simulink model "RealLifeTrainModel"  (R2024a)
settings: Solver=ode1  StartTime=0.0  StopTime=Inf  FixedStep=0.001  RelTol=1e-3
PostLoadFcn:
  | , if any(exist('dsrtsu_mdlpostloadfcn', 'file') ~= 0), dsrtsu_mdlpostloadfcn('Execute', bdroot); end,
InitFcn:
  | , if any(exist('rtifpga_mdlclblib', 'file') ~= 0), rtifpga_mdlclblib('Init', bdroot); end,
undefined symbols (not defined in the file): DiscIntNeverNeededParam
libraries: deeplib x29, svdutilitieslib x28, simulink x8, eeGeneralControl x8, rti1202lib_adc_class1 x6, rti1202serlib x5, spsEdgeDetectorLib x5, rtiemclib x2, rti1202lib_dac_class1 x1
(part 6 of 8)

== matlab function RealLifeTrainModel/ContractionMetricFilterSystem3/CalcK/IndidualGrad6/Policy_SS1/Denormalize_Policy ==
  data: u input; y output
function y = fcn(u)

max_Fload =  569.629505294963
min_Fload = -610.339671010468

max_Fhyd = 729.261146885585
min_Fhyd = -777.489547410502

max_DFload = 123011.265014651
min_DFload = -142353.177843906

max_DFhyd = 219994.429294316
min_DFhyd = -270882.694509076

max_Pa = 12037835.3221229
min_Pa = 1849925.22965178

max_Pb = 14831789.6053956
min_Pb = 2808786.27887814

max_x = 0.082368752
min_x = 0.01990812

max_Dx = 0.682789396628826
min_Dx = -0.578996654196926

out = [1,1,1,1,1,1,1,1,1]

out(1) = (u(1))*(max_Fhyd - min_Fhyd) + min_Fhyd;

out(2) = (u(2))*(max_DFhyd - min_DFhyd) + min_DFhyd;

out(3) = (u(3))*(max_Fload - min_Fload) + min_Fload;

out(4) = (u(4))*(max_DFload - min_DFload) + min_DFload;

out(5) = (u(5))*(max_Pa - min_Pa) + min_Pa;

out(6) = (u(6))*(max_Pb - min_Pb) + min_Pb;

out(7) = (u(7))*(max_x - min_x) + min_x;

out(8) = (u(8))*(max_Dx - min_Dx) + min_Dx;

out(9) = (u(9))*(max_Fload - min_Fload) + min_Fload;


y = out;

== matlab function RealLifeTrainModel/ContractionMetricFilterSystem3/CalcK/IndidualGrad6/Policy_SS1/FLcontroller1 ==
  data: pid input; y output; f input; g input; dFref input; d input; flag_start input
function y = fcn(pid,f,g,dFref,d,flag_start)

if flag_start == 1
    y = (dFref + pid - f)/g - d;
else 
    y = 1;
end

== matlab function RealLifeTrainModel/ContractionMetricFilterSystem3/CalcK/IndidualGrad6/Policy_SS1/FunctionCalculateHydModel1 ==
  data: ixv input; f output; Pn input; Qn input; Un input; Vpl input; Ps input; Pt input; L_cyl input; Aa input; alfa input; c1 input; c2 input; Be input; flag_start input; data input; g output; force output
function [f,g,force] = fcn(ixv,Pn,Qn,Un,Vpl,Ps,Pt,L_cyl,Aa,alfa,c1,c2,Be,flag_start,data)
force = 0
if flag_start == 1
    Pa = data(5)
    Pb = data(6)
    xp = data(7)
    xpd = data(8)
    force = data(3)

    Kv = Qn/(Un*sqrt(Pn/2));
    
    Va = Vpl + Aa*xp;
    Vb = Vpl + (L_cyl - xp)*alfa*Aa;

    if(ixv >= 0)
        g = Be*Aa*Kv*( sign(Ps-Pa)*sqrt(abs(Ps-Pa))/Va + alfa*sign(Pb-Pt)*sqrt(abs(Pb-Pt))/Vb);
    else
        g = Be*Aa*Kv*( sign(Pa-Pt)*sqrt(abs(Pa-Pt))/Va + alfa*sign(Ps-Pb)*sqrt(abs(Ps-Pb))/Vb);
    end
    
    %g1 = Be*Aa*Kv*( sign(Ps-Pa)*sqrt(abs(Ps-Pa))/Va + alfa*sign(Pb-Pt)*sqrt(abs(Pb-Pt))/Vb);
    %g2 = Be*Aa*Kv*( sign(Pa-Pt)*sqrt(abs(Pa-Pt))/Va + alfa*sign(Ps-Pb)*sqrt(abs(Ps-Pb))/Vb);
    %g = (g1 + g2)/2;

    f = -Be*Aa^2*(((alfa)^2)/Vb + 1/Va)*xpd;
    
    g = c2*g;
    f = c1*f;
    
else
    f = 1;
    g = 1;
end

== matlab function RealLifeTrainModel/DisturbanceEstimationPhase2 ==
  data: g input; lambda input; F input; d output; z input; dist_model input; gain1 input; gain2 input; Fmenos_z input; intFmenos_z input; flag_start input; intintFmenos_z input; gain3 input
function d = fcn(g,lambda,F,z,dist_model,gain1,gain2,Fmenos_z,intFmenos_z,flag_start,intintFmenos_z,gain3)

if(flag_start == 1)
    if(dist_model == 0)
        d = (z);
    elseif (dist_model == 1)
        d = (z + lambda*F/(g));
    elseif (dist_model == 2)
        d = gain1*Fmenos_z + gain2*(intFmenos_z) + gain3*intintFmenos_z;
    else
        d = (z + lambda*F)/g;
    end
    
else
    d = 0;
end

== matlab function RealLifeTrainModel/ContractionMetricFilterSystem3/CalcK/IndidualGrad6/Policy_SS1/Policy ==
  data: u input; y output
function y = fcn(u)

y = (u)/2 + 0.5;

== matlab function RealLifeTrainModel/ContractionMetricFilterSystem3/CalcK/IndidualGrad6/Policy_SS1/SmoothFnc1 ==
  data: u input; y output; smooth input
function y = fcn(u,smooth)
persistent last_value;

if(isempty(last_value))
    last_value = 0
end

y = smooth*last_value + (1 - smooth)*u
last_value = u

== matlab function RealLifeTrainModel/ContractionMetricFilterSystem3/CalcK/IndidualGrad7/MATLAB Function2 ==
  data: u input; y output; pos input
function y = fcn(u,pos)

a = [0,0,0,0,0,0,0,0,0]

a(pos) = u

y = a;

== matlab function RealLifeTrainModel/ContractionMetricFilterSystem3/CalcK/IndidualGrad7/MATLAB Function5 ==
  data: u1 input; y output; u2 input; const input
function y = fcn(u1,u2,const)

y = (u1 - u2)/(const);

== matlab function RealLifeTrainModel/ContractionMetricFilterSystem3/CalcK/IndidualGrad7/Policy_SS1/Denormalize_Policy ==
  data: u input; y output
function y = fcn(u)

max_Fload =  569.629505294963
min_Fload = -610.339671010468

max_Fhyd = 729.261146885585
min_Fhyd = -777.489547410502

max_DFload = 123011.265014651
min_DFload = -142353.177843906

max_DFhyd = 219994.429294316
min_DFhyd = -270882.694509076

max_Pa = 12037835.3221229
min_Pa = 1849925.22965178

max_Pb = 14831789.6053956
min_Pb = 2808786.27887814

max_x = 0.082368752
min_x = 0.01990812

max_Dx = 0.682789396628826
min_Dx = -0.578996654196926

out = [1,1,1,1,1,1,1,1,1]

out(1) = (u(1))*(max_Fhyd - min_Fhyd) + min_Fhyd;

out(2) = (u(2))*(max_DFhyd - min_DFhyd) + min_DFhyd;

out(3) = (u(3))*(max_Fload - min_Fload) + min_Fload;

out(4) = (u(4))*(max_DFload - min_DFload) + min_DFload;

out(5) = (u(5))*(max_Pa - min_Pa) + min_Pa;

out(6) = (u(6))*(max_Pb - min_Pb) + min_Pb;

out(7) = (u(7))*(max_x - min_x) + min_x;

out(8) = (u(8))*(max_Dx - min_Dx) + min_Dx;

out(9) = (u(9))*(max_Fload - min_Fload) + min_Fload;


y = out;

== matlab function RealLifeTrainModel/ContractionMetricFilterSystem3/CalcK/IndidualGrad7/Policy_SS1/FLcontroller1 ==
  data: pid input; y output; f input; g input; dFref input; d input; flag_start input
function y = fcn(pid,f,g,dFref,d,flag_start)

if flag_start == 1
    y = (dFref + pid - f)/g - d;
else 
    y = 1;
end

== matlab function RealLifeTrainModel/ContractionMetricFilterSystem3/CalcK/IndidualGrad7/Policy_SS1/FunctionCalculateHydModel1 ==
  data: ixv input; f output; Pn input; Qn input; Un input; Vpl input; Ps input; Pt input; L_cyl input; Aa input; alfa input; c1 input; c2 input; Be input; flag_start input; data input; g output; force output
function [f,g,force] = fcn(ixv,Pn,Qn,Un,Vpl,Ps,Pt,L_cyl,Aa,alfa,c1,c2,Be,flag_start,data)
force = 0
if flag_start == 1
    Pa = data(5)
    Pb = data(6)
    xp = data(7)
    xpd = data(8)
    force = data(3)

    Kv = Qn/(Un*sqrt(Pn/2));
    
    Va = Vpl + Aa*xp;
    Vb = Vpl + (L_cyl - xp)*alfa*Aa;

    if(ixv >= 0)
        g = Be*Aa*Kv*( sign(Ps-Pa)*sqrt(abs(Ps-Pa))/Va + alfa*sign(Pb-Pt)*sqrt(abs(Pb-Pt))/Vb);
    else
        g = Be*Aa*Kv*( sign(Pa-Pt)*sqrt(abs(Pa-Pt))/Va + alfa*sign(Ps-Pb)*sqrt(abs(Ps-Pb))/Vb);
    end
    
    %g1 = Be*Aa*Kv*( sign(Ps-Pa)*sqrt(abs(Ps-Pa))/Va + alfa*sign(Pb-Pt)*sqrt(abs(Pb-Pt))/Vb);
    %g2 = Be*Aa*Kv*( sign(Pa-Pt)*sqrt(abs(Pa-Pt))/Va + alfa*sign(Ps-Pb)*sqrt(abs(Ps-Pb))/Vb);
    %g = (g1 + g2)/2;

    f = -Be*Aa^2*(((alfa)^2)/Vb + 1/Va)*xpd;
    
    g = c2*g;
    f = c1*f;
    
else
    f = 1;
    g = 1;
end

== matlab function RealLifeTrainModel/ContractionMetricFilterSystem3/CalcK/IndidualGrad7/Policy_SS1/Policy ==
  data: u input; y output
function y = fcn(u)

y = (u)/2 + 0.5;

== matlab function RealLifeTrainModel/ContractionMetricFilterSystem3/CalcK/IndidualGrad7/Policy_SS1/SmoothFnc1 ==
  data: u input; y output; smooth input
function y = fcn(u,smooth)
persistent last_value;

if(isempty(last_value))
    last_value = 0
end

y = smooth*last_value + (1 - smooth)*u
last_value = u

== matlab function RealLifeTrainModel/ContractionMetricFilterSystem3/CalcK/Policy_SS1/Denormalize_Policy ==
  data: u input; y output
function y = fcn(u)

max_Fload =  569.629505294963
min_Fload = -610.339671010468

max_Fhyd = 729.261146885585
min_Fhyd = -777.489547410502

max_DFload = 123011.265014651
min_DFload = -142353.177843906

max_DFhyd = 219994.429294316
min_DFhyd = -270882.694509076

max_Pa = 12037835.3221229
min_Pa = 1849925.22965178

max_Pb = 14831789.6053956
min_Pb = 2808786.27887814

max_x = 0.082368752
min_x = 0.01990812

max_Dx = 0.682789396628826
min_Dx = -0.578996654196926

out = [1,1,1,1,1,1,1,1,1]

out(1) = (u(1))*(max_Fhyd - min_Fhyd) + min_Fhyd;

out(2) = (u(2))*(max_DFhyd - min_DFhyd) + min_DFhyd;

out(3) = (u(3))*(max_Fload - min_Fload) + min_Fload;

out(4) = (u(4))*(max_DFload - min_DFload) + min_DFload;

out(5) = (u(5))*(max_Pa - min_Pa) + min_Pa;

out(6) = (u(6))*(max_Pb - min_Pb) + min_Pb;

out(7) = (u(7))*(max_x - min_x) + min_x;

out(8) = (u(8))*(max_Dx - min_Dx) + min_Dx;

out(9) = (u(9))*(max_Fload - min_Fload) + min_Fload;


y = out;

== matlab function RealLifeTrainModel/ContractionMetricFilterSystem3/CalcK/Policy_SS1/FLcontroller1 ==
  data: pid input; y output; f input; g input; dFref input; d input; flag_start input
function y = fcn(pid,f,g,dFref,d,flag_start)

if flag_start == 1
    y = (dFref + pid - f)/g - d;
else 
    y = 1;
end

== matlab function RealLifeTrainModel/ContractionMetricFilterSystem3/CalcK/Policy_SS1/FunctionCalculateHydModel1 ==
  data: ixv input; f output; Pn input; Qn input; Un input; Vpl input; Ps input; Pt input; L_cyl input; Aa input; alfa input; c1 input; c2 input; Be input; flag_start input; data input; g output; force output
function [f,g,force] = fcn(ixv,Pn,Qn,Un,Vpl,Ps,Pt,L_cyl,Aa,alfa,c1,c2,Be,flag_start,data)
force = 0
if flag_start == 1
    Pa = data(5)
    Pb = data(6)
    xp = data(7)
    xpd = data(8)
    force = data(3)

    Kv = Qn/(Un*sqrt(Pn/2));
    
    Va = Vpl + Aa*xp;
    Vb = Vpl + (L_cyl - xp)*alfa*Aa;

    if(ixv >= 0)
        g = Be*Aa*Kv*( sign(Ps-Pa)*sqrt(abs(Ps-Pa))/Va + alfa*sign(Pb-Pt)*sqrt(abs(Pb-Pt))/Vb);
    else
        g = Be*Aa*Kv*( sign(Pa-Pt)*sqrt(abs(Pa-Pt))/Va + alfa*sign(Ps-Pb)*sqrt(abs(Ps-Pb))/Vb);
    end
    
    %g1 = Be*Aa*Kv*( sign(Ps-Pa)*sqrt(abs(Ps-Pa))/Va + alfa*sign(Pb-Pt)*sqrt(abs(Pb-Pt))/Vb);
    %g2 = Be*Aa*Kv*( sign(Pa-Pt)*sqrt(abs(Pa-Pt))/Va + alfa*sign(Ps-Pb)*sqrt(abs(Ps-Pb))/Vb);
    %g = (g1 + g2)/2;

    f = -Be*Aa^2*(((alfa)^2)/Vb + 1/Va)*xpd;
    
    g = c2*g;
    f = c1*f;
    
else
    f = 1;
    g = 1;
end

== matlab function RealLifeTrainModel/ContractionMetricFilterSystem3/CalcK/Policy_SS1/Policy ==
  data: u input; y output
function y = fcn(u)

y = (u)/2 + 0.5;

== matlab function RealLifeTrainModel/ContractionMetricFilterSystem3/CalcK/Policy_SS1/SmoothFnc1 ==
  data: u input; y output; smooth input
function y = fcn(u,smooth)
persistent last_value;

if(isempty(last_value))
    last_value = 0
end

y = smooth*last_value + (1 - smooth)*u
last_value = u

== matlab function RealLifeTrainModel/ContractionMetricFilterSystem3/Calc_A_B/Calc_A_Grad/DynamicsConvert ==
  data: x input; dstate output; y_model input; useDerivative input
function dstate = DynamicsConvert(x, y_model, useDerivative)
%#codegen
% Uses ONLY the first 8 elements of x (and y_model).
% Fixed sample time dt = 0.001 s.
% Output: 8x1, same class as x (single/double).

% Force column shape
x       = x(:);
y_model = y_model(:);

% Sanity checks
assert(numel(x) >= 8 && numel(y_model) >= 8);

% Slice first 8
x8 = x(1:8);
y8 = y_model(1:8);

% Compute in double, then cast back to 'like x'
xd  = double(x8);
yd  = double(y8);
dtd = 1e-3;  % fixed dt = 0.001 s

if logical(useDerivative)
    % y_model is xdot (use first 8 components)
    tmp = yd;               % 8x1
else
    % y_model is next-state (use first 8 components) -> derivative
    tmp = (yd - xd) ./ dtd; % 8x1
end

% Final: cast to match x's class and enforce 8x1 shape
dstate = cast(tmp, 'like', x8);
dstate = reshape(dstate, 8, 1);

== matlab function RealLifeTrainModel/ContractionMetricFilterSystem3/Calc_A_B/Calc_A_Grad/IndidualGrad1/DynamicsConvert ==
  data: x input; dstate output; y_model input; useDerivative input
function dstate = DynamicsConvert(x, y_model, useDerivative)
%#codegen
% Uses ONLY the first 8 elements of x (and y_model).
% Fixed sample time dt = 0.001 s.
% Output: 8x1, same class as x (single/double).

% Force column shape
x       = x(:);
y_model = y_model(:);

% Sanity checks
assert(numel(x) >= 8 && numel(y_model) >= 8);

% Slice first 8
x8 = x(1:8);
y8 = y_model(1:8);

% Compute in double, then cast back to 'like x'
xd  = double(x8);
yd  = double(y8);
dtd = 1e-3;  % fixed dt = 0.001 s

if logical(useDerivative)
    % y_model is xdot (use first 8 components)
    tmp = yd;               % 8x1
else
    % y_model is next-state (use first 8 components) -> derivative
    tmp = (yd - xd) ./ dtd; % 8x1
end

% Final: cast to match x's class and enforce 8x1 shape
dstate = cast(tmp, 'like', x8);
dstate = reshape(dstate, 8, 1);

== matlab function RealLifeTrainModel/ContractionMetricFilterSystem3/Calc_A_B/Calc_A_Grad/IndidualGrad1/MATLAB Function2 ==
  data: u input; y output; pos input
function y = fcn(u,pos)

a = [0,0,0,0,0,0,0,0,0]

a(pos) = u

y = a;

== matlab function RealLifeTrainModel/ContractionMetricFilterSystem3/Calc_A_B/Calc_A_Grad/IndidualGrad1/MATLAB Function5 ==
  data: u1 input; y output; u2 input; const input
function y = fcn(u1,u2,const)

y = (u1 - u2)/(const);

== matlab function RealLifeTrainModel/ADCReadToNewtons_Hyd ==
  data: u input; y output
function y = fcn(u)
u = mean(u);
LOADCELL_5000_RANGE = 5000.0;
voltage = u;


tau_sensors_nofilt = (voltage)*LOADCELL_5000_RANGE;


y = tau_sensors_nofilt;

== matlab function RealLifeTrainModel/ContractionMetricFilterSystem3/Calc_A_B/Calc_A_Grad/IndidualGrad1/SubsystemModel/Denormalize ==
  data: u input; y output
function y = fcn(u)
u = u/2  + 0.5
y = u;

== matlab function RealLifeTrainModel/ContractionMetricFilterSystem3/Calc_A_B/Calc_A_Grad/IndidualGrad1/SubsystemModel/Normalize ==
  data: u input; y output
function y = fcn(u)
u = 2*u - 1
y = u;

== matlab function RealLifeTrainModel/ContractionMetricFilterSystem3/Calc_A_B/Calc_A_Grad/IndidualGrad10/DynamicsConvert ==
  data: x input; dstate output; y_model input; useDerivative input
function dstate = DynamicsConvert(x, y_model, useDerivative)
%#codegen
% Uses ONLY the first 8 elements of x (and y_model).
% Fixed sample time dt = 0.001 s.
% Output: 8x1, same class as x (single/double).

% Force column shape
x       = x(:);
y_model = y_model(:);

% Sanity checks
assert(numel(x) >= 8 && numel(y_model) >= 8);

% Slice first 8
x8 = x(1:8);
y8 = y_model(1:8);

% Compute in double, then cast back to 'like x'
xd  = double(x8);
yd  = double(y8);
dtd = 1e-3;  % fixed dt = 0.001 s

if logical(useDerivative)
    % y_model is xdot (use first 8 components)
    tmp = yd;               % 8x1
else
    % y_model is next-state (use first 8 components) -> derivative
    tmp = (yd - xd) ./ dtd; % 8x1
end

% Final: cast to match x's class and enforce 8x1 shape
dstate = cast(tmp, 'like', x8);
dstate = reshape(dstate, 8, 1);

== matlab function RealLifeTrainModel/ContractionMetricFilterSystem3/Calc_A_B/Calc_A_Grad/IndidualGrad10/MATLAB Function2 ==
  data: u input; y output; pos input
function y = fcn(u,pos)

a = [0,0,0,0,0,0,0,0,0]

a(pos) = u

y = a;

== matlab function RealLifeTrainModel/ContractionMetricFilterSystem3/Calc_A_B/Calc_A_Grad/IndidualGrad10/MATLAB Function5 ==
  data: u1 input; y output; u2 input; const input
function y = fcn(u1,u2,const)

y = (u1 - u2)/(const);

== matlab function RealLifeTrainModel/ContractionMetricFilterSystem3/Calc_A_B/Calc_A_Grad/IndidualGrad10/SubsystemModel/Denormalize ==
  data: u input; y output
function y = fcn(u)
u = u/2  + 0.5
y = u;

== matlab function RealLifeTrainModel/ContractionMetricFilterSystem3/Calc_A_B/Calc_A_Grad/IndidualGrad10/SubsystemModel/Normalize ==
  data: u input; y output
function y = fcn(u)
u = 2*u - 1
y = u;

== matlab function RealLifeTrainModel/ContractionMetricFilterSystem3/Calc_A_B/Calc_A_Grad/IndidualGrad2/DynamicsConvert ==
  data: x input; dstate output; y_model input; useDerivative input
function dstate = DynamicsConvert(x, y_model, useDerivative)
%#codegen
% Uses ONLY the first 8 elements of x (and y_model).
% Fixed sample time dt = 0.001 s.
% Output: 8x1, same class as x (single/double).

% Force column shape
x       = x(:);
y_model = y_model(:);

% Sanity checks
assert(numel(x) >= 8 && numel(y_model) >= 8);

% Slice first 8
x8 = x(1:8);
y8 = y_model(1:8);

% Compute in double, then cast back to 'like x'
xd  = double(x8);
yd  = double(y8);
dtd = 1e-3;  % fixed dt = 0.001 s

if logical(useDerivative)
    % y_model is xdot (use first 8 components)
    tmp = yd;               % 8x1
else
    % y_model is next-state (use first 8 components) -> derivative
    tmp = (yd - xd) ./ dtd; % 8x1
end

% Final: cast to match x's class and enforce 8x1 shape
dstate = cast(tmp, 'like', x8);
dstate = reshape(dstate, 8, 1);

== matlab function RealLifeTrainModel/ContractionMetricFilterSystem3/Calc_A_B/Calc_A_Grad/IndidualGrad2/MATLAB Function2 ==
  data: u input; y output; pos input
function y = fcn(u,pos)

a = [0,0,0,0,0,0,0,0,0]

a(pos) = u

y = a;

== matlab function RealLifeTrainModel/ADCReadToPressure ==
  data: u input; y output
function y = fcn(u)
u = mean(u);
max_press = 250*100000;%pa
voltage = ((u));


pressure_pa = (voltage)*max_press;


y = pressure_pa;

== matlab function RealLifeTrainModel/ContractionMetricFilterSystem3/Calc_A_B/Calc_A_Grad/IndidualGrad2/MATLAB Function5 ==
  data: u1 input; y output; u2 input; const input
function y = fcn(u1,u2,const)

y = (u1 - u2)/(const);

== matlab function RealLifeTrainModel/ContractionMetricFilterSystem3/Calc_A_B/Calc_A_Grad/IndidualGrad2/SubsystemModel/Denormalize ==
  data: u input; y output
function y = fcn(u)
u = u/2  + 0.5
y = u;

== matlab function RealLifeTrainModel/ContractionMetricFilterSystem3/Calc_A_B/Calc_A_Grad/IndidualGrad2/SubsystemModel/Normalize ==
  data: u input; y output
function y = fcn(u)
u = 2*u - 1
y = u;

== matlab function RealLifeTrainModel/ContractionMetricFilterSystem3/Calc_A_B/Calc_A_Grad/IndidualGrad3/DynamicsConvert ==
  data: x input; dstate output; y_model input; useDerivative input
function dstate = DynamicsConvert(x, y_model, useDerivative)
%#codegen
% Uses ONLY the first 8 elements of x (and y_model).
% Fixed sample time dt = 0.001 s.
% Output: 8x1, same class as x (single/double).

% Force column shape
x       = x(:);
y_model = y_model(:);

% Sanity checks
assert(numel(x) >= 8 && numel(y_model) >= 8);

% Slice first 8
x8 = x(1:8);
y8 = y_model(1:8);

% Compute in double, then cast back to 'like x'
xd  = double(x8);
yd  = double(y8);
dtd = 1e-3;  % fixed dt = 0.001 s

if logical(useDerivative)
    % y_model is xdot (use first 8 components)
    tmp = yd;               % 8x1
else
    % y_model is next-state (use first 8 components) -> derivative
    tmp = (yd - xd) ./ dtd; % 8x1
end

% Final: cast to match x's class and enforce 8x1 shape
dstate = cast(tmp, 'like', x8);
dstate = reshape(dstate, 8, 1);

== matlab function RealLifeTrainModel/ContractionMetricFilterSystem3/Calc_A_B/Calc_A_Grad/IndidualGrad3/MATLAB Function2 ==
  data: u input; y output; pos input
function y = fcn(u,pos)

a = [0,0,0,0,0,0,0,0,0]

a(pos) = u

y = a;

== matlab function RealLifeTrainModel/ContractionMetricFilterSystem3/Calc_A_B/Calc_A_Grad/IndidualGrad3/MATLAB Function5 ==
  data: u1 input; y output; u2 input; const input
function y = fcn(u1,u2,const)

y = (u1 - u2)/(const);

== matlab function RealLifeTrainModel/ContractionMetricFilterSystem3/Calc_A_B/Calc_A_Grad/IndidualGrad3/SubsystemModel/Denormalize ==
  data: u input; y output
function y = fcn(u)
u = u/2  + 0.5
y = u;

== matlab function RealLifeTrainModel/ContractionMetricFilterSystem3/Calc_A_B/Calc_A_Grad/IndidualGrad3/SubsystemModel/Normalize ==
  data: u input; y output
function y = fcn(u)
u = 2*u - 1
y = u;

== matlab function RealLifeTrainModel/ADCReadToNewtons_Load ==
  data: u input; y output
function y = fcn(u)
u = mean(u);
LOADCELL_5000_RANGE = 5000.0;
voltage = u;


tau_sensors_nofilt = (voltage)*LOADCELL_5000_RANGE;


y = tau_sensors_nofilt;

== matlab function RealLifeTrainModel/ContractionMetricFilterSystem3/Calc_A_B/Calc_A_Grad/IndidualGrad4/DynamicsConvert ==
  data: x input; dstate output; y_model input; useDerivative input
function dstate = DynamicsConvert(x, y_model, useDerivative)
%#codegen
% Uses ONLY the first 8 elements of x (and y_model).
% Fixed sample time dt = 0.001 s.
% Output: 8x1, same class as x (single/double).

% Force column shape
x       = x(:);
y_model = y_model(:);

% Sanity checks
assert(numel(x) >= 8 && numel(y_model) >= 8);

% Slice first 8
x8 = x(1:8);
y8 = y_model(1:8);

% Compute in double, then cast back to 'like x'
xd  = double(x8);
yd  = double(y8);
dtd = 1e-3;  % fixed dt = 0.001 s

if logical(useDerivative)
    % y_model is xdot (use first 8 components)
    tmp = yd;               % 8x1
else
    % y_model is next-state (use first 8 components) -> derivative
    tmp = (yd - xd) ./ dtd; % 8x1
end

% Final: cast to match x's class and enforce 8x1 shape
dstate = cast(tmp, 'like', x8);
dstate = reshape(dstate, 8, 1);

== matlab function RealLifeTrainModel/ContractionMetricFilterSystem3/Calc_A_B/Calc_A_Grad/IndidualGrad4/MATLAB Function2 ==
  data: u input; y output; pos input
function y = fcn(u,pos)

a = [0,0,0,0,0,0,0,0,0]

a(pos) = u

y = a;

== matlab function RealLifeTrainModel/ContractionMetricFilterSystem3/Calc_A_B/Calc_A_Grad/IndidualGrad4/MATLAB Function5 ==
  data: u1 input; y output; u2 input; const input
function y = fcn(u1,u2,const)

y = (u1 - u2)/(const);

== matlab function RealLifeTrainModel/ContractionMetricFilterSystem3/Calc_A_B/Calc_A_Grad/IndidualGrad4/SubsystemModel/Denormalize ==
  data: u input; y output
function y = fcn(u)
u = u/2  + 0.5
y = u;

== matlab function RealLifeTrainModel/ContractionMetricFilterSystem3/Calc_A_B/Calc_A_Grad/IndidualGrad4/SubsystemModel/Normalize ==
  data: u input; y output
function y = fcn(u)
u = 2*u - 1
y = u;

== matlab function RealLifeTrainModel/ContractionMetricFilterSystem3/Calc_A_B/Calc_A_Grad/IndidualGrad5/DynamicsConvert ==
  data: x input; dstate output; y_model input; useDerivative input
function dstate = DynamicsConvert(x, y_model, useDerivative)
%#codegen
% Uses ONLY the first 8 elements of x (and y_model).
% Fixed sample time dt = 0.001 s.
% Output: 8x1, same class as x (single/double).

% Force column shape
x       = x(:);
y_model = y_model(:);

% Sanity checks
assert(numel(x) >= 8 && numel(y_model) >= 8);

% Slice first 8
x8 = x(1:8);
y8 = y_model(1:8);

% Compute in double, then cast back to 'like x'
xd  = double(x8);
yd  = double(y8);
dtd = 1e-3;  % fixed dt = 0.001 s

if logical(useDerivative)
    % y_model is xdot (use first 8 components)
    tmp = yd;               % 8x1
else
    % y_model is next-state (use first 8 components) -> derivative
    tmp = (yd - xd) ./ dtd; % 8x1
end

% Final: cast to match x's class and enforce 8x1 shape
dstate = cast(tmp, 'like', x8);
dstate = reshape(dstate, 8, 1);

== matlab function RealLifeTrainModel/ContractionMetricFilterSystem3/Calc_A_B/Calc_A_Grad/IndidualGrad5/MATLAB Function2 ==
  data: u input; y output; pos input
function y = fcn(u,pos)

a = [0,0,0,0,0,0,0,0,0]

a(pos) = u

y = a;

== matlab function RealLifeTrainModel/ContractionMetricFilterSystem3/Calc_A_B/Calc_A_Grad/IndidualGrad5/MATLAB Function5 ==
  data: u1 input; y output; u2 input; const input
function y = fcn(u1,u2,const)

y = (u1 - u2)/(const);

== matlab function RealLifeTrainModel/ContractionMetricFilterSystem3/Calc_A_B/Calc_A_Grad/IndidualGrad5/SubsystemModel/Denormalize ==
  data: u input; y output
function y = fcn(u)
u = u/2  + 0.5
y = u;

== matlab function RealLifeTrainModel/ADCReadToPressure1 ==
  data: u input; y output
function y = fcn(u)
u = mean(u);
max_press = 250*100000;%pa
voltage = ((u));


pressure_pa = (voltage)*max_press;


y = pressure_pa;

== matlab function RealLifeTrainModel/ContractionMetricFilterSystem3/Calc_A_B/Calc_A_Grad/IndidualGrad5/SubsystemModel/Normalize ==
  data: u input; y output
function y = fcn(u)
u = 2*u - 1
y = u;

== matlab function RealLifeTrainModel/ContractionMetricFilterSystem3/Calc_A_B/Calc_A_Grad/IndidualGrad6/DynamicsConvert ==
  data: x input; dstate output; y_model input; useDerivative input
function dstate = DynamicsConvert(x, y_model, useDerivative)
%#codegen
% Uses ONLY the first 8 elements of x (and y_model).
% Fixed sample time dt = 0.001 s.
% Output: 8x1, same class as x (single/double).

% Force column shape
x       = x(:);
y_model = y_model(:);

% Sanity checks
assert(numel(x) >= 8 && numel(y_model) >= 8);

% Slice first 8
x8 = x(1:8);
y8 = y_model(1:8);

% Compute in double, then cast back to 'like x'
xd  = double(x8);
yd  = double(y8);
dtd = 1e-3;  % fixed dt = 0.001 s

if logical(useDerivative)
    % y_model is xdot (use first 8 components)
    tmp = yd;               % 8x1
else
    % y_model is next-state (use first 8 components) -> derivative
    tmp = (yd - xd) ./ dtd; % 8x1
end

% Final: cast to match x's class and enforce 8x1 shape
dstate = cast(tmp, 'like', x8);
dstate = reshape(dstate, 8, 1);

== matlab function RealLifeTrainModel/ContractionMetricFilterSystem3/Calc_A_B/Calc_A_Grad/IndidualGrad6/MATLAB Function2 ==
  data: u input; y output; pos input
function y = fcn(u,pos)

a = [0,0,0,0,0,0,0,0,0]

a(pos) = u

y = a;

== matlab function RealLifeTrainModel/ContractionMetricFilterSystem3/Calc_A_B/Calc_A_Grad/IndidualGrad6/MATLAB Function5 ==
  data: u1 input; y output; u2 input; const input
function y = fcn(u1,u2,const)

y = (u1 - u2)/(const);

== matlab function RealLifeTrainModel/ContractionMetricFilterSystem3/Calc_A_B/Calc_A_Grad/IndidualGrad6/SubsystemModel/Denormalize ==
  data: u input; y output
function y = fcn(u)
u = u/2  + 0.5
y = u;

== matlab function RealLifeTrainModel/ContractionMetricFilterSystem3/Calc_A_B/Calc_A_Grad/IndidualGrad6/SubsystemModel/Normalize ==
  data: u input; y output
function y = fcn(u)
u = 2*u - 1
y = u;

== matlab function RealLifeTrainModel/ContractionMetricFilterSystem3/Calc_A_B/Calc_A_Grad/IndidualGrad7/DynamicsConvert ==
  data: x input; dstate output; y_model input; useDerivative input
function dstate = DynamicsConvert(x, y_model, useDerivative)
%#codegen
% Uses ONLY the first 8 elements of x (and y_model).
% Fixed sample time dt = 0.001 s.
% Output: 8x1, same class as x (single/double).

% Force column shape
x       = x(:);
y_model = y_model(:);

% Sanity checks
assert(numel(x) >= 8 && numel(y_model) >= 8);

% Slice first 8
x8 = x(1:8);
y8 = y_model(1:8);

% Compute in double, then cast back to 'like x'
xd  = double(x8);
yd  = double(y8);
dtd = 1e-3;  % fixed dt = 0.001 s

if logical(useDerivative)
    % y_model is xdot (use first 8 components)
    tmp = yd;               % 8x1
else
    % y_model is next-state (use first 8 components) -> derivative
    tmp = (yd - xd) ./ dtd; % 8x1
end

% Final: cast to match x's class and enforce 8x1 shape
dstate = cast(tmp, 'like', x8);
dstate = reshape(dstate, 8, 1);

== matlab function RealLifeTrainModel/ContractionMetricFilterSystem3/Calc_A_B/Calc_A_Grad/IndidualGrad7/MATLAB Function2 ==
  data: u input; y output; pos input
function y = fcn(u,pos)

a = [0,0,0,0,0,0,0,0,0]

a(pos) = u

y = a;

== matlab function RealLifeTrainModel/ContractionMetricFilterSystem3/Calc_A_B/Calc_A_Grad/IndidualGrad7/MATLAB Function5 ==
  data: u1 input; y output; u2 input; const input
function y = fcn(u1,u2,const)

y = (u1 - u2)/(const);

== matlab function RealLifeTrainModel/ADCReadToPressure2 ==
  data: u input; y output
function y = fcn(u)
u = mean(u);
max_press = 250*100000;%pa
voltage = ((u));


pressure_pa = (voltage)*max_press;


y = pressure_pa;

== matlab function RealLifeTrainModel/ContractionMetricFilterSystem3/Calc_A_B/Calc_A_Grad/IndidualGrad7/SubsystemModel/Denormalize ==
  data: u input; y output
function y = fcn(u)
u = u/2  + 0.5
y = u;

== matlab function RealLifeTrainModel/ContractionMetricFilterSystem3/Calc_A_B/Calc_A_Grad/IndidualGrad7/SubsystemModel/Normalize ==
  data: u input; y output
function y = fcn(u)
u = 2*u - 1
y = u;

== matlab function RealLifeTrainModel/ContractionMetricFilterSystem3/Calc_A_B/Calc_A_Grad/IndidualGrad8/DynamicsConvert1 ==
  data: x input; dstate output; y_model input; useDerivative input
function dstate = DynamicsConvert(x, y_model, useDerivative)
%#codegen
% Uses ONLY the first 8 elements of x (and y_model).
% Fixed sample time dt = 0.001 s.
% Output: 8x1, same class as x (single/double).

% Force column shape
x       = x(:);
y_model = y_model(:);

% Sanity checks
assert(numel(x) >= 8 && numel(y_model) >= 8);

% Slice first 8
x8 = x(1:8);
y8 = y_model(1:8);

% Compute in double, then cast back to 'like x'
xd  = double(x8);
yd  = double(y8);
dtd = 1e-3;  % fixed dt = 0.001 s

if logical(useDerivative)
    % y_model is xdot (use first 8 components)
    tmp = yd;               % 8x1
else
    % y_model is next-state (use first 8 components) -> derivative
    tmp = (yd - xd) ./ dtd; % 8x1
end

% Final: cast to match x's class and enforce 8x1 shape
dstate = cast(tmp, 'like', x8);
dstate = reshape(dstate, 8, 1);

== matlab function RealLifeTrainModel/ContractionMetricFilterSystem3/Calc_A_B/Calc_A_Grad/IndidualGrad8/MATLAB Function2 ==
  data: u input; y output; pos input
function y = fcn(u,pos)

a = [0,0,0,0,0,0,0,0,0]

a(pos) = u

y = a;

== matlab function RealLifeTrainModel/ContractionMetricFilterSystem3/Calc_A_B/Calc_A_Grad/IndidualGrad8/MATLAB Function5 ==
  data: u1 input; y output; u2 input; const input
function y = fcn(u1,u2,const)

y = (u1 - u2)/(const);

== matlab function RealLifeTrainModel/ContractionMetricFilterSystem3/Calc_A_B/Calc_A_Grad/IndidualGrad8/SubsystemModel/Denormalize ==
  data: u input; y output
function y = fcn(u)
u = u/2  + 0.5
y = u;

== matlab function RealLifeTrainModel/ContractionMetricFilterSystem3/Calc_A_B/Calc_A_Grad/IndidualGrad8/SubsystemModel/Normalize ==
  data: u input; y output
function y = fcn(u)
u = 2*u - 1
y = u;

== matlab function RealLifeTrainModel/ContractionMetricFilterSystem3/Calc_A_B/Calc_A_Grad/SubsystemModel/Denormalize ==
  data: u input; y output
function y = fcn(u)
u = u/2  + 0.5
y = u;

== matlab function RealLifeTrainModel/ContractionMetricFilterSystem3/Calc_A_B/Calc_A_Grad/SubsystemModel/Normalize ==
  data: u input; y output
function y = fcn(u)
u = 2*u - 1
y = u;

== matlab function RealLifeTrainModel/ADCReadToPressure3 ==
  data: u input; y output
function y = fcn(u)
u = mean(u);
max_press = 250*100000;%pa
voltage = ((u));


pressure_pa = (voltage)*max_press;


y = pressure_pa;

== matlab function RealLifeTrainModel/ContractionMetricFilterSystem3/ConvertMatrix ==
  data: M_flat input; M output
function M = fcn(M_flat)
%#codegen
coder.inline('always');

n = 8;
assert(isvector(M_flat) && numel(M_flat) == n*n);

% Ensure type/shape
M_flat = single(M_flat(:));      % 64x1 single

% If input was Python-row-major flattened:
Mraw = reshape(M_flat, n, n).';  % 8x8 single (transpose = row->col major)


% SPD enforcement
eps_pd = single(1e-3);
M = (Mraw.' * Mraw) + eps_pd * eye(n, 'like', Mraw);
end

== matlab function RealLifeTrainModel/ContractionMetricFilterSystem3/MATLAB Function1 ==
  data: x input; u_filtered output; ref input; u_nom input; A input; B input; K input; M_curr_flat input; M_prev_flat input; dt input; task_dim input; row_major input; td_is_zero_based input; eps_pd input; cert_val output; is_active output; a_val output; b_val output; use_A_transpose input; du_out output; Mdot input; lambda_val input
function [u_filtered, cert_val, is_active, a_val, b_val, du_out] = ...
    qp_filter_projected_deltaU( ...
        x, ref, u_nom, ...
        A, B, K, ...
        M_curr_flat, M_prev_flat, ...
        dt, task_dim,    ...
        row_major, td_is_zero_based, eps_pd, use_A_transpose,Mdot,lambda_val) %#codegen
% Closed-form QP: min 0.5*||du||^2 s.t. a'*du <= b, with u_filt = u_nom + du
% Works for m >= 1 (vector control). Codegen-safe for Simulink.

% ---------- local flags / defaults ----------
if nargin < 12 || isempty(row_major),        row_major = true;  end
if nargin < 13 || isempty(td_is_zero_based), td_is_zero_based = true; end
if nargin < 14 || isempty(eps_pd),           eps_pd = single(1e-3);   end
if nargin < 15 || isempty(use_A_transpose),  use_A_transpose = false; end

rowMajor    = (row_major ~= 0);
tdZeroBased = (td_is_zero_based ~= 0);
useAT       = (use_A_transpose ~= 0);

% ---------- sizes ----------
nM = int32(numel(M_curr_flat));
n  = 8
% Shapes
x_m = reshape(x, [], 1);           % n x 1
A_m = reshape(A, n, n);            % n x n
B_m = reshape(B, n, []);           % n x m
K_m = reshape(K, [], n);           % m x n
m   = size(B_m, 2);

% ---------- metric reshape (+ row/col-major fix) ----------
M_curr = M_curr_flat

% ---------- Mdot from previous ----------
%if dt > 0
%    M_dot = (M_curr - M_prev) ./ cast(dt, 'like', M_curr);
%else
%    M_dot = zeros(n, n, 'like', M_curr);
%end
M_dot = Mdot;

% ---------- ABK (optionally with A') ----------
A_use = A_m; if useAT, A_use = A_m.'; end

if rowMajor 
    M_curr = M_curr.'; 
    M_dot = M_dot.'
end

ABK = A_use + B_m * K_m;                % n x n

% ---------- contraction matrix ----------
sym = M_curr * ABK;  sym = sym + sym.';   % symmetrized M*ABK
C   = M_dot + sym + (2 * cast(lambda_val, 'like', M_curr)) * M_curr;

% ---------- contracting direction v ----------
if tdZeroBased
    td = int32(task_dim) + 1;    % Python 0-based -> MATLAB 1-based
else
    td = int32(task_dim);
end
td = max(1, min(td, n));

v = zeros(n,1,'like',M_curr);
v(td,1) = cast(x_m(td,1) - cast(ref,'like',x_m), 'like', M_curr);

% ---------- certificate & half-space ----------
cert_val = cast(v' * C * v, 'like', u_nom);             % 1x1

a_row = 2*(v' * (M_curr * B_m));                    % 1 x m
b_val = cast(-(v' * C * v), 'like', u_nom);             % scalar

% ---------- closed-form projection in Δu-space ----------
a_col  = cast(a_row.', 'like', u_nom);                  % m x 1
anorm2 = max(cast(1e-12, 'like', u_nom), sum(a_col .* a_col));  % scalar

if b_val >= 0
    du = zeros(m, 1, 'like', u_nom);                    % inactive
    active = 0;
else
    du = (b_val / anorm2) * a_col;                      % active
    active = 1;
end

if du > eps_pd
    du = eps_pd
end
if du < -eps_pd
    du = -eps_pd
end

u_filtered = u_nom + du;                                 % m x 1
is_active  = double(active);                             % codegen-friendly (0/1)
a_val      = a_col;                                      % return as column (m x 1)
du_out     = du;                                         % expose Δu for debugging
end

== matlab function RealLifeTrainModel/ContractionMetricFilterSystem3/MATLAB Function3 ==
  data: a_flat input; M output; eps input
function M = build_metric(a_flat, eps) %#codegen
% a_flat: 64x1 or 1x64 (fixed size). Output M: 8x8.
% eps: scalar (e.g., 1e-3). Set data type to match your pipeline.

% ---- compile-time constants ----
n = coder.const(8);

% ---- ensure column vector, preserve type ----
a_flat = reshape(a_flat, [], 1);

% NOTE on layout:
% PyTorch flattens in row-major. MATLAB reshape is column-major.
% Using transpose below aligns PyTorch's layout with MATLAB's.
A = reshape(a_flat, [n, n]).';   % 8x8

% ---- compute M = A' * A + eps * I ----
M = A.' * A;
M = M + cast(eps, 'like', a_flat) * eye(n, 'like', a_flat);
end

== matlab function RealLifeTrainModel/ContractionMetricFilterSystem3/Mdot_subsystem/ConvertMatrix ==
  data: M_flat input; M output
function M = fcn(M_flat)
%#codegen
coder.inline('always');

n = 8;
assert(isvector(M_flat) && numel(M_flat) == n*n);

% Ensure type/shape
M_flat = single(M_flat(:));      % 64x1 single

% If input was Python-row-major flattened:
Mraw = reshape(M_flat, n, n).';  % 8x8 single (transpose = row->col major)

% SPD enforcement
eps_pd = single(1e-3);
M = (Mraw.' * Mraw) + eps_pd * eye(n, 'like', Mraw);
end

== matlab function RealLifeTrainModel/ContractionMetricFilterSystem3/Mdot_subsystem/IndidualGrad1/ConvertMatrix ==
  data: M_flat input; M output
function M = fcn(M_flat)
%#codegen
coder.inline('always');

n = 8;
assert(isvector(M_flat) && numel(M_flat) == n*n);

% Ensure type/shape
M_flat = single(M_flat(:));      % 64x1 single

% If input was Python-row-major flattened:
Mraw = reshape(M_flat, n, n).';  % 8x8 single (transpose = row->col major)

% SPD enforcement
eps_pd = single(1e-3);
M = (Mraw.' * Mraw) + eps_pd * eye(n, 'like', Mraw);
end

== matlab function RealLifeTrainModel/ContractionMetricFilterSystem3/Mdot_subsystem/IndidualGrad1/MATLAB Function2 ==
  data: u input; y output; pos input
function y = fcn(u,pos)

a = [0,0,0,0,0,0,0,0]

a(pos) = u

y = a;

== matlab function RealLifeTrainModel/ContractionMetricFilterSystem3/Mdot_subsystem/IndidualGrad1/MATLAB Function5 ==
  data: u1 input; y output; u2 input; const input
function y = fcn(u1,u2,const)

y = (u1 - u2)/(const);

== matlab function RealLifeTrainModel/MATLAB Function1 ==
  data: edge input; y output; last_value input; v output; last_value_counter input; last_value_recording input; x output; last_value_disturb input; last_value_z input; w output; e output
function [y,v,x,w,e] = fcn(edge,last_value,last_value_counter,last_value_recording,last_value_disturb,last_value_z)
y = 1;
if(edge == 1)
    y = 0;
    v = 0;
    x = 0;
    w = 0;
    e = 0;
else
    y = last_value;
    v = last_value_counter;
    x = last_value_recording;
    w = last_value_disturb;
    e = last_value_z;
end

== matlab function RealLifeTrainModel/ContractionMetricFilterSystem3/Mdot_subsystem/IndidualGrad10/ConvertMatrix ==
  data: M_flat input; M output
function M = fcn(M_flat)
%#codegen
coder.inline('always');

n = 8;
assert(isvector(M_flat) && numel(M_flat) == n*n);

% Ensure type/shape
M_flat = single(M_flat(:));      % 64x1 single

% If input was Python-row-major flattened:
Mraw = reshape(M_flat, n, n).';  % 8x8 single (transpose = row->col major)

% SPD enforcement
eps_pd = single(1e-3);
M = (Mraw.' * Mraw) + eps_pd * eye(n, 'like', Mraw);
end

== matlab function RealLifeTrainModel/ContractionMetricFilterSystem3/Mdot_subsystem/IndidualGrad10/MATLAB Function2 ==
  data: u input; y output; pos input
function y = fcn(u,pos)

a = [0,0,0,0,0,0,0,0]

a(pos) = u

y = a;

== matlab function RealLifeTrainModel/ContractionMetricFilterSystem3/Mdot_subsystem/IndidualGrad10/MATLAB Function5 ==
  data: u1 input; y output; u2 input; const input
function y = fcn(u1,u2,const)

y = (u1 - u2)/(const);

== matlab function RealLifeTrainModel/ContractionMetricFilterSystem3/Mdot_subsystem/IndidualGrad2/ConvertMatrix ==
  data: M_flat input; M output
function M = fcn(M_flat)
%#codegen
coder.inline('always');

n = 8;
assert(isvector(M_flat) && numel(M_flat) == n*n);

% Ensure type/shape
M_flat = single(M_flat(:));      % 64x1 single

% If input was Python-row-major flattened:
Mraw = reshape(M_flat, n, n).';  % 8x8 single (transpose = row->col major)

% SPD enforcement
eps_pd = single(1e-3);
M = (Mraw.' * Mraw) + eps_pd * eye(n, 'like', Mraw);
end

== matlab function RealLifeTrainModel/ContractionMetricFilterSystem3/Mdot_subsystem/IndidualGrad2/MATLAB Function2 ==
  data: u input; y output; pos input
function y = fcn(u,pos)

a = [0,0,0,0,0,0,0,0]

a(pos) = u

y = a;

== matlab function RealLifeTrainModel/ContractionMetricFilterSystem3/Mdot_subsystem/IndidualGrad2/MATLAB Function5 ==
  data: u1 input; y output; u2 input; const input
function y = fcn(u1,u2,const)

y = (u1 - u2)/(const);

== matlab function RealLifeTrainModel/ContractionMetricFilterSystem3/Mdot_subsystem/IndidualGrad3/ConvertMatrix ==
  data: M_flat input; M output
function M = fcn(M_flat)
%#codegen
coder.inline('always');

n = 8;
assert(isvector(M_flat) && numel(M_flat) == n*n);

% Ensure type/shape
M_flat = single(M_flat(:));      % 64x1 single

% If input was Python-row-major flattened:
Mraw = reshape(M_flat, n, n).';  % 8x8 single (transpose = row->col major)

% SPD enforcement
eps_pd = single(1e-3);
M = (Mraw.' * Mraw) + eps_pd * eye(n, 'like', Mraw);
end

== matlab function RealLifeTrainModel/ContractionMetricFilterSystem3/Mdot_subsystem/IndidualGrad3/MATLAB Function2 ==
  data: u input; y output; pos input
function y = fcn(u,pos)

a = [0,0,0,0,0,0,0,0]

a(pos) = u

y = a;

== matlab function RealLifeTrainModel/ContractionMetricFilterSystem3/Mdot_subsystem/IndidualGrad3/MATLAB Function5 ==
  data: u1 input; y output; u2 input; const input
function y = fcn(u1,u2,const)

y = (u1 - u2)/(const);

== matlab function RealLifeTrainModel/ContractionMetricFilterSystem3/Mdot_subsystem/IndidualGrad4/ConvertMatrix ==
  data: M_flat input; M output
function M = fcn(M_flat)
%#codegen
coder.inline('always');

n = 8;
assert(isvector(M_flat) && numel(M_flat) == n*n);

% Ensure type/shape
M_flat = single(M_flat(:));      % 64x1 single

% If input was Python-row-major flattened:
Mraw = reshape(M_flat, n, n).';  % 8x8 single (transpose = row->col major)

% SPD enforcement
eps_pd = single(1e-3);
M = (Mraw.' * Mraw) + eps_pd * eye(n, 'like', Mraw);
end

== matlab function RealLifeTrainModel/ContractionMetricFilterSystem3/Mdot_subsystem/IndidualGrad4/MATLAB Function2 ==
  data: u input; y output; pos input
function y = fcn(u,pos)

a = [0,0,0,0,0,0,0,0]

a(pos) = u

y = a;

== matlab function RealLifeTrainModel/ContractionMetricFilterSystem3/Mdot_subsystem/IndidualGrad4/MATLAB Function5 ==
  data: u1 input; y output; u2 input; const input
function y = fcn(u1,u2,const)

y = (u1 - u2)/(const);

== matlab function RealLifeTrainModel/ContractionMetricFilterSystem3/Mdot_subsystem/IndidualGrad5/ConvertMatrix ==
  data: M_flat input; M output
function M = fcn(M_flat)
%#codegen
coder.inline('always');

n = 8;
assert(isvector(M_flat) && numel(M_flat) == n*n);

% Ensure type/shape
M_flat = single(M_flat(:));      % 64x1 single

% If input was Python-row-major flattened:
Mraw = reshape(M_flat, n, n).';  % 8x8 single (transpose = row->col major)

% SPD enforcement
eps_pd = single(1e-3);
M = (Mraw.' * Mraw) + eps_pd * eye(n, 'like', Mraw);
end

== matlab function RealLifeTrainModel/ContractionMetricFilterSystem3/Mdot_subsystem/IndidualGrad5/MATLAB Function2 ==
  data: u input; y output; pos input
function y = fcn(u,pos)

a = [0,0,0,0,0,0,0,0]

a(pos) = u

y = a;

== matlab function RealLifeTrainModel/ContractionMetricFilterSystem3/Mdot_subsystem/IndidualGrad5/MATLAB Function5 ==
  data: u1 input; y output; u2 input; const input
function y = fcn(u1,u2,const)

y = (u1 - u2)/(const);

== matlab function RealLifeTrainModel/ContractionMetricFilterSystem3/Mdot_subsystem/IndidualGrad6/ConvertMatrix ==
  data: M_flat input; M output
function M = fcn(M_flat)
%#codegen
coder.inline('always');

n = 8;
assert(isvector(M_flat) && numel(M_flat) == n*n);

% Ensure type/shape
M_flat = single(M_flat(:));      % 64x1 single

% If input was Python-row-major flattened:
Mraw = reshape(M_flat, n, n).';  % 8x8 single (transpose = row->col major)

% SPD enforcement
eps_pd = single(1e-3);
M = (Mraw.' * Mraw) + eps_pd * eye(n, 'like', Mraw);
end

== matlab function RealLifeTrainModel/ContractionMetricFilterSystem3/Mdot_subsystem/IndidualGrad6/MATLAB Function2 ==
  data: u input; y output; pos input
function y = fcn(u,pos)

a = [0,0,0,0,0,0,0,0]

a(pos) = u

y = a;

== matlab function RealLifeTrainModel/ContractionMetricFilterSystem3/Mdot_subsystem/IndidualGrad6/MATLAB Function5 ==
  data: u1 input; y output; u2 input; const input
function y = fcn(u1,u2,const)

y = (u1 - u2)/(const);

== matlab function RealLifeTrainModel/ContractionMetricFilterSystem3/Mdot_subsystem/IndidualGrad7/ConvertMatrix ==
  data: M_flat input; M output
function M = fcn(M_flat)
%#codegen
coder.inline('always');

n = 8;
assert(isvector(M_flat) && numel(M_flat) == n*n);

% Ensure type/shape
M_flat = single(M_flat(:));      % 64x1 single

% If input was Python-row-major flattened:
Mraw = reshape(M_flat, n, n).';  % 8x8 single (transpose = row->col major)

% SPD enforcement
eps_pd = single(1e-3);
M = (Mraw.' * Mraw) + eps_pd * eye(n, 'like', Mraw);
end

== matlab function RealLifeTrainModel/ContractionMetricFilterSystem3/Mdot_subsystem/IndidualGrad7/MATLAB Function2 ==
  data: u input; y output; pos input
function y = fcn(u,pos)

a = [0,0,0,0,0,0,0,0]

a(pos) = u

y = a;

== matlab function RealLifeTrainModel/StartStopRecordingController ==
  data: start_signal_value input; start_signal_value_update output; recording_signal_value input; counter_value input; recording_signal_value_update output; counter_value_update output; start_time input; number_experiments input; experiment_time_value input; time input; last_disturb input; last_z input; last_disturb_update output; last_z_update output
function [start_signal_value_update,recording_signal_value_update,counter_value_update,last_disturb_update,last_z_update] = fcn(start_signal_value, ...
    recording_signal_value,counter_value,start_time,number_experiments,experiment_time_value,time,last_disturb,last_z)



if(start_signal_value == 0)
    recording_signal_value = 0;
    counter_value = 0;
elseif(start_signal_value == 1)

    if(counter_value == number_experiments)
        start_signal_value = 0;
    elseif(recording_signal_value == 0 & (((time - start_time) - experiment_time_value) > 0.2 | counter_value == 0))
        recording_signal_value = 1;
        last_disturb = 0;
        last_z = 0;
    elseif((time - start_time) > experiment_time_value & recording_signal_value == 1)
        recording_signal_value = 0;
        counter_value = counter_value + 1;
    end 

end

last_disturb_update = last_disturb;
last_z_update = last_z;
start_signal_value_update = start_signal_value;
recording_signal_value_update = recording_signal_value;
counter_value_update = counter_value;

== matlab function RealLifeTrainModel/ContractionMetricFilterSystem3/Mdot_subsystem/IndidualGrad7/MATLAB Function5 ==
  data: u1 input; y output; u2 input; const input
function y = fcn(u1,u2,const)

y = (u1 - u2)/(const);

== matlab function RealLifeTrainModel/ContractionMetricFilterSystem3/NormalizeMetric_1 ==
  data: u input; y output
function y = fcn(u)

max_Fload =  569.629505294963
min_Fload = -610.339671010468

max_Fhyd = 729.261146885585
min_Fhyd = -777.489547410502

max_DFload = 123011.265014651
min_DFload = -142353.177843906

max_DFhyd = 219994.429294316
min_DFhyd = -270882.694509076

max_Pa = 12037835.3221229
min_Pa = 1849925.22965178

max_Pb = 14831789.6053956
min_Pb = 2808786.27887814

max_x = 0.082368752
min_x = 0.01990812

max_Dx = 0.682789396628826
min_Dx = -0.578996654196926

out = [1,1,1,1,1,1,1,1]

out(1) = (u(1) - min_Fhyd)/(max_Fhyd - min_Fhyd);
out(2) = (u(2) - min_DFhyd)/(max_DFhyd - min_DFhyd);
out(3) = (u(3) - min_Fload)/(max_Fload - min_Fload);
out(4) = (u(4) - min_DFload)/(max_DFload - min_DFload);
out(5) = (u(5) - min_Pa)/(max_Pa - min_Pa);
out(6) = (u(6) - min_Pb)/(max_Pb - min_Pb);
out(7) = (u(7) - min_x)/(max_x - min_x);
out(8) = (u(8) - min_Dx)/(max_Dx - min_Dx);



y = out;

== matlab function RealLifeTrainModel/ContractionMetricFilterSystem3/NormalizeMetric_2 ==
  data: u input; y output
function y = fcn(u)

max_Fload =  569.629505294963
min_Fload = -610.339671010468

max_Fhyd = 729.261146885585
min_Fhyd = -777.489547410502

max_DFload = 123011.265014651
min_DFload = -142353.177843906

max_DFhyd = 219994.429294316
min_DFhyd = -270882.694509076

max_Pa = 12037835.3221229
min_Pa = 1849925.22965178

max_Pb = 14831789.6053956
min_Pb = 2808786.27887814

max_x = 0.082368752
min_x = 0.01990812

max_Dx = 0.682789396628826
min_Dx = -0.578996654196926

out = [1]


out(1) = (u(1) - min_Fload)/(max_Fload - min_Fload);




y = out;

== matlab function RealLifeTrainModel/ContractionMetricFilterSystem3/NormalizeMetric_8 ==
  data: u input; y output
function y = fcn(u)
max_Fload =  569.629505294963
min_Fload = -610.339671010468

max_Fhyd = 729.261146885585
min_Fhyd = -777.489547410502

max_DFload = 123011.265014651
min_DFload = -142353.177843906

max_DFhyd = 219994.429294316
min_DFhyd = -270882.694509076

max_Pa = 12037835.3221229
min_Pa = 1849925.22965178

max_Pb = 14831789.6053956
min_Pb = 2808786.27887814

max_x = 0.082368752
min_x = 0.01990812

max_Dx = 0.682789396628826
min_Dx = -0.578996654196926

out = [1,1,1,1,1,1,1,1]

out(1) = (u(1) - min_Fhyd)/(max_Fhyd - min_Fhyd);
out(2) = (u(2) - min_DFhyd)/(max_DFhyd - min_DFhyd);
out(3) = (u(3) - min_Fload)/(max_Fload - min_Fload);
out(4) = (u(4) - min_DFload)/(max_DFload - min_DFload);
out(5) = (u(5) - min_Pa)/(max_Pa - min_Pa);
out(6) = (u(6) - min_Pb)/(max_Pb - min_Pb);
out(7) = (u(7) - min_x)/(max_x - min_x);
out(8) = (u(8) - min_Dx)/(max_Dx - min_Dx);




y = out;

== matlab function RealLifeTrainModel/ContractionMetricFilterSystem3/NormalizeMetric_9 ==
  data: u input; y output
function y = fcn(u)
max_Fload =  569.629505294963
min_Fload = -610.339671010468

max_Fhyd = 729.261146885585
min_Fhyd = -777.489547410502

max_DFload = 123011.265014651
min_DFload = -142353.177843906

max_DFhyd = 219994.429294316
min_DFhyd = -270882.694509076

max_Pa = 12037835.3221229
min_Pa = 1849925.22965178

max_Pb = 14831789.6053956
min_Pb = 2808786.27887814

max_x = 0.082368752
min_x = 0.01990812

max_Dx = 0.682789396628826
min_Dx = -0.578996654196926

out = [1,1,1,1,1,1,1,1,1]

out(1) = (u(1) - min_Fhyd)/(max_Fhyd - min_Fhyd);
out(2) = (u(2) - min_DFhyd)/(max_DFhyd - min_DFhyd);
out(3) = (u(3) - min_Fload)/(max_Fload - min_Fload);
out(4) = (u(4) - min_DFload)/(max_DFload - min_DFload);
out(5) = (u(5) - min_Pa)/(max_Pa - min_Pa);
out(6) = (u(6) - min_Pb)/(max_Pb - min_Pb);
out(7) = (u(7) - min_x)/(max_x - min_x);
out(8) = (u(8) - min_Dx)/(max_Dx - min_Dx);
out(9) = (u(9) - min_Fload)/(max_Fload - min_Fload);



y = out;
